simulink model "loop"  (Simulink 8.5)
settings: Solver=VariableStepDiscrete  StartTime=0.0  StopTime=50  RelTol=1e-3
settings Model: Creator=a  LastModifiedBy=rootprfl
settings DebuggingCC: FcnCallInpInsideContextMsg=EnableAllAsWarning
settings SimEventsCC: propDiagStatOutput=1

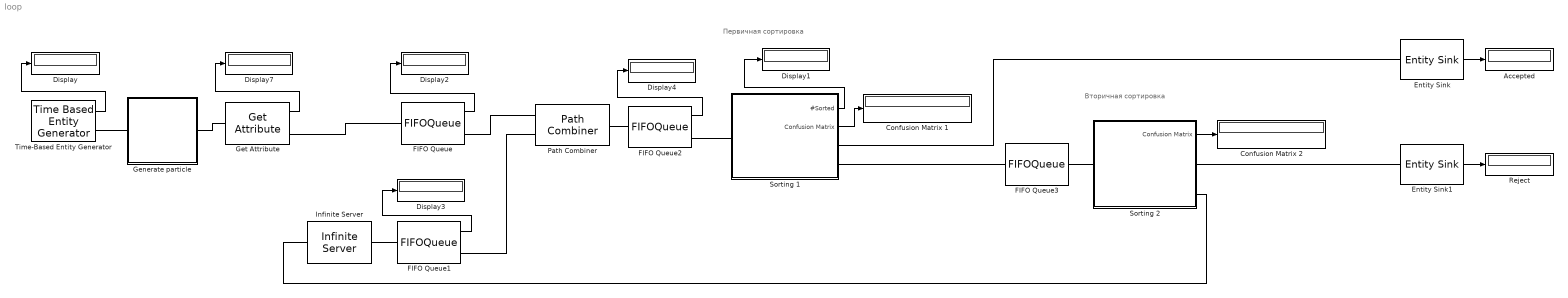
== system loop ==
  note: Вторичная сортировка
  note: Первичная сортировка
  Accepted : Display
  Confusion Matrix 1 : Display
  Confusion Matrix 2 : Display
  Display{,1..4,7} (6 alike) : Display
      Display7 settings: Decimation=3
  Entity Sink : EntitySink  StatNumberArrived=on
  Entity Sink1 : EntitySink  StatNumberArrived=on
  FIFO Queue : FIFOQueue  Capacity=10000  StatNumberDeparted=on
  FIFO Queue1 : FIFOQueue  Capacity=10000  StatNumberDeparted=on
  FIFO Queue2 : FIFOQueue  Capacity=10000  StatNumberDeparted=on
  FIFO Queue3 : FIFOQueue  Capacity=10000
  Generate particle : Subsystem
  Get Attribute : GetAttribute  AttributeName=label  EvaluatedDefaultAttributeValue={ []}
      settings: OutputPortMap=o1
  Infinite Server : InfiniteServer  ServiceTime=10
  Path Combiner : PathCombiner  NumberInputPorts=2  InputPortPrecedence=Equiprobable
  Reject : Display
  Sorting 1 : Subsystem
  Sorting 2 : Subsystem
  Time-Based Entity Generator : TimeBasedEntityGenerator  Distribution=Uniform  GenerateEntityAtSimulationStart=off  StatNumberDeparted=on
  wires:
  Time-Based Entity Generator/1 -> Display/1
  FIFO Queue/1 -> Display2/1
  FIFO Queue1/1 -> Display3/1
  FIFO Queue2/1 -> Display4/1
  Entity Sink/1 -> Accepted/1
  Entity Sink1/1 -> Reject/1
  Get Attribute/1 -> Display7/1
  Sorting 1/1("#Sorted ") -> Display1/1
  Sorting 2/1(Confusion Matrix) -> Confusion Matrix 2/1
  Sorting 1/2(Confusion Matrix) -> Confusion Matrix 1/1
  connections:
  Get Attribute/RConn1 -- FIFO Queue/LConn1
  FIFO Queue1/RConn1 -- Path Combiner/LConn2
  FIFO Queue/RConn1 -- Path Combiner/LConn1
  Infinite Server/RConn1 -- FIFO Queue1/LConn1
  Path Combiner/RConn1 -- FIFO Queue2/LConn1
  Generate particle/RConn1 -- Get Attribute/LConn1
  Time-Based Entity Generator/RConn1 -- Generate particle/LConn1
  Sorting 1/RConn1 -- Entity Sink/LConn1
  FIFO Queue2/RConn1 -- Sorting 1/LConn1
  Sorting 1/RConn2 -- FIFO Queue3/LConn1
  FIFO Queue3/RConn1 -- Sorting 2/LConn1
  Entity Sink1/LConn1 -- Sorting 2/RConn1
  Infinite Server/LConn1 -- Sorting 2/RConn2

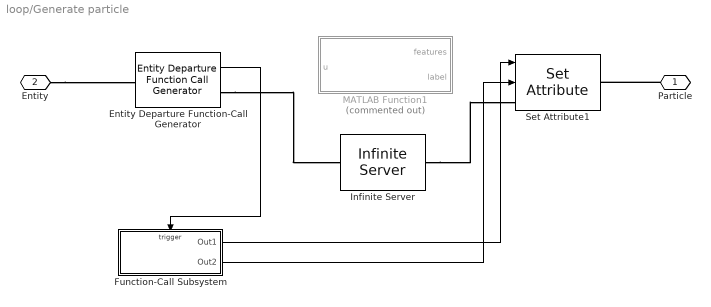
== system loop/Generate particle ==
  Entity Departure Function-Call Generator : EntityDepartureFunctionCallGenerator
  Function-Call Subsystem : Subsystem  TreatAsAtomicUnit=on
  Infinite Server : InfiniteServer
  MATLAB Function1 : MATLAB Function  Commented=on  TreatAsAtomicUnit=on
  Set Attribute1 : SetAttribute  AttributeName=features|label  AttributeFrom=Signal port|Signal port  AttributeValue=[0 0]|1  AttributeTreatAsVector=1|1  EvaluatedAttributeValue={ [];[]}
      settings: InputPortMap=u0,u1
  Particle : PMIOPort  Port=1  Side=Right
  Entity : PMIOPort  Port=2  Side=Left
  wires:
  Function-Call Subsystem/1(Out1) -> Set Attribute1/1
  Function-Call Subsystem/2(Out2) -> Set Attribute1/2
  Entity Departure Function-Call Generator/1 -> Function-Call Subsystem/Trigger
  connections:
  Particle/RConn1 -- Set Attribute1/RConn1
  Entity/RConn1 -- Entity Departure Function-Call Generator/LConn1
  Entity Departure Function-Call Generator/RConn1 -- Infinite Server/LConn1
  Infinite Server/RConn1 -- Set Attribute1/LConn1

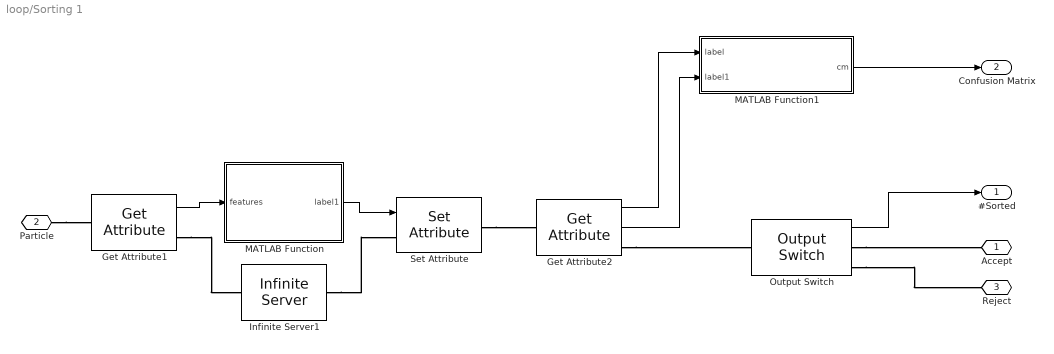
== system loop/Sorting 1 ==
  Get Attribute1 : GetAttribute  AttributeName=features  EvaluatedDefaultAttributeValue={ []}
      settings: OutputPortMap=o1
  Get Attribute2 : GetAttribute  AttributeName=label|label1  AttributeMissing=Error|Error  AttributeDefaultValue=1|1  AttributeTreatAsVector=1|1  AttributeSendTiming=After entity departure|After entity departure  EvaluatedDefaultAttributeValue={ [];[]}
      settings: OutputPortMap=o1,o2
  Infinite Server1 : InfiniteServer
  MATLAB Function : MATLAB Function  TreatAsAtomicUnit=on
  MATLAB Function1 : MATLAB Function  TreatAsAtomicUnit=on
  Output Switch : OutputSwitch  NumberOutputPorts=2  SwitchingCriterion=From attribute  AttributeName=label1  StatNumberDeparted=on
  Set Attribute : SetAttribute  AttributeName=label1  AttributeFrom=Signal port  EvaluatedAttributeValue={ []}
  Accept : PMIOPort  Port=1  Side=Right
  Particle : PMIOPort  Port=2  Side=Left
  Reject : PMIOPort  Port=3  Side=Right
  "#Sorted " : Outport
  Confusion Matrix : Outport  Port=2
  wires:
  Output Switch/1 -> "#Sorted "/1
  Get Attribute1/1 -> MATLAB Function/1(features)
  MATLAB Function/1(label1) -> Set Attribute/1
  Get Attribute2/1 -> MATLAB Function1/1(label)
  Get Attribute2/2 -> MATLAB Function1/2(label1)
  MATLAB Function1/1(cm) -> Confusion Matrix/1
  connections:
  Particle/RConn1 -- Get Attribute1/LConn1
  Output Switch/RConn2 -- Reject/RConn1
  Output Switch/RConn1 -- Accept/RConn1
  Infinite Server1/RConn1 -- Set Attribute/LConn1
  Get Attribute1/RConn1 -- Infinite Server1/LConn1
  Set Attribute/RConn1 -- Get Attribute2/LConn1
  Get Attribute2/RConn1 -- Output Switch/LConn1

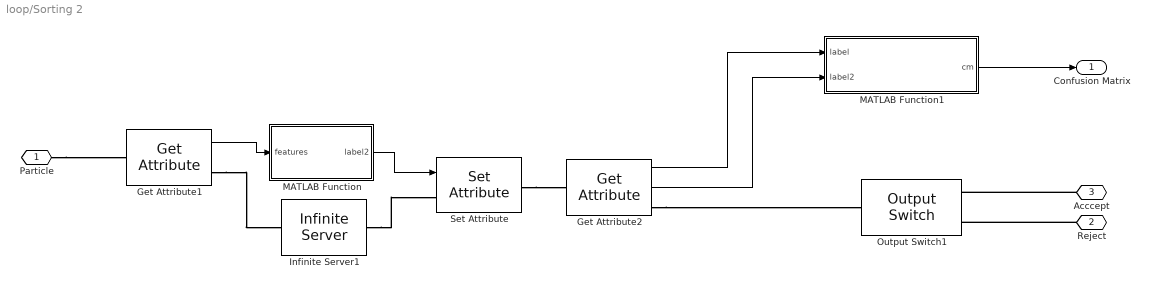
== system loop/Sorting 2 ==
  Get Attribute1 : GetAttribute  AttributeName=features  EvaluatedDefaultAttributeValue={ []}
      settings: OutputPortMap=o1
  Get Attribute2 : GetAttribute  AttributeName=label|label2  AttributeMissing=Error|Error  AttributeDefaultValue=1|1  AttributeTreatAsVector=1|1  AttributeSendTiming=After entity departure|After entity departure  EvaluatedDefaultAttributeValue={ [];[]}
      settings: OutputPortMap=o1,o2
  Infinite Server1 : InfiniteServer
  MATLAB Function : MATLAB Function  TreatAsAtomicUnit=on
  MATLAB Function1 : MATLAB Function  TreatAsAtomicUnit=on
  Output Switch1 : OutputSwitch  NumberOutputPorts=2  SwitchingCriterion=From attribute  InitialSeed=5677  AttributeName=label2
  Set Attribute : SetAttribute  AttributeName=label2  AttributeFrom=Signal port  EvaluatedAttributeValue={ []}
  Particle : PMIOPort  Port=1  Side=Left
  Reject : PMIOPort  Port=2  Side=Right
  Acccept : PMIOPort  Port=3  Side=Right
  Confusion Matrix : Outport
  wires:
  Get Attribute1/1 -> MATLAB Function/1(features)
  MATLAB Function/1(label2) -> Set Attribute/1
  Get Attribute2/1 -> MATLAB Function1/1(label)
  Get Attribute2/2 -> MATLAB Function1/2(label2)
  MATLAB Function1/1(cm) -> Confusion Matrix/1
  connections:
  Reject/RConn1 -- Output Switch1/RConn2
  Get Attribute1/RConn1 -- Infinite Server1/LConn1
  Particle/RConn1 -- Get Attribute1/LConn1
  Infinite Server1/RConn1 -- Set Attribute/LConn1
  Set Attribute/RConn1 -- Get Attribute2/LConn1
  Acccept/RConn1 -- Output Switch1/RConn1
  Get Attribute2/RConn1 -- Output Switch1/LConn1

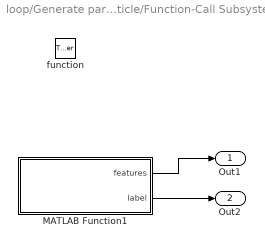
== system loop/Generate particle/Function-Call Subsystem ==
  function : TriggerPort  TriggerType=function-call
  MATLAB Function1 : MATLAB Function  TreatAsAtomicUnit=on
  Out1 : Outport
  Out2 : Outport  Port=2
  wires:
  MATLAB Function1/1(features) -> Out1/1
  MATLAB Function1/2(label) -> Out2/1

== matlab function Generate particle/MATLAB Function1 ==
  data: u input double; features output double; Params parameter double; label output double
function [features, label] = GenFeatures(u,Params)
%#codegen
[features, protonum] = clonesample(Params.Xsrc,1);
label = Params.Lsrc(protonum);

== matlab function Generate particle/Function-Call Subsystem/MATLAB Function1 ==
  data: features output double; Params parameter double; label output double
function [features, label] = GenFeatures(Params)
%#codegen
[features, protonum] = clonesample(Params.Xsrc,1);
label = Params.Lsrc(protonum);

== matlab function Sorting 1/MATLAB Function ==
  data: features input double; label1 output double; Params parameter double
function label1  = SortIt(features,Params)%function [label1, fp1, fn1] = SortIt(features,Params)
%#codegen
% label1 = 1 if model < 0, 
% label1 = 2 if model > 0
% fp1 = 1 if particle is classified as false positive, 0 otherwise
% fn1 = 1 if particle is classified as false negative, 0 otherwise

label1 = double(Params.B1(1) + features*Params.B1(2:end) > 0)+1;
%fp1 = double((label1 == 1) & (label == 2));
%fn1 = double((label1 == 2) & (label == 1));

== matlab function Sorting 2/MATLAB Function ==
  data: features input double; label2 output double; Params parameter double
function label2  = SortIt(features,Params)%function [label2, fp2, fn2] = SortIt(features,Params)
%#codegen%
% label2 = 1 if model < 0, 
% label2 = 2 if model > 0
% fp2 = 1 if particle is classified as false positive, 0 otherwise
% fn2 = 1 if particle is classified as false negative, 0 otherwise

label2 = double(Params.B2(1) + features*Params.B2(2:end) > 0)+1;
%fp2 = double((label2 == 1) & (label == 2));
%fn2 = double((label2 == 2) & (label == 1));

== matlab function Sorting 2/MATLAB Function1 ==
  data: label input double; cm output double; label2 input double
function cm = ConfusionMatrix(label,label2)
%#codegen
persistent CM

if isempty(CM)
    CM=zeros(2,2);
end

CM(1,1) = CM(1,1) + (label==1 & label2==1);
CM(1,2) = CM(1,2) + (label==1 & label2==2);
CM(2,1) = CM(2,1) + (label==2 & label2==1);
CM(2,2) = CM(2,2) + (label==2 & label2==2);

cm = CM;

== matlab function Sorting 1/MATLAB Function1 ==
  data: label input double; cm output double; label1 input double
function cm = ConfusionMatrix(label,label1)
%#codegen
persistent CM

if isempty(CM)
    CM=zeros(2,2);
end

CM(1,1) = CM(1,1) + (label==1 & label1==1);
CM(1,2) = CM(1,2) + (label==1 & label1==2);
CM(2,1) = CM(2,1) + (label==2 & label1==1);
CM(2,2) = CM(2,2) + (label==2 & label1==2);

cm = CM;
